simulink model "RLcircuit"  (R2018a)
settings: Solver=ode45  StartTime=0.0  StopTime=5.0  RelTol=1e-3
values from neighbouring files (symbols this model uses):
  R = sqrt(x.^2+y.^2)    [ex2_5.m]
undefined symbols (not defined in the file or in its folder): L
settings Model: Creator=Guestmit  LastModifiedBy=Guestmit

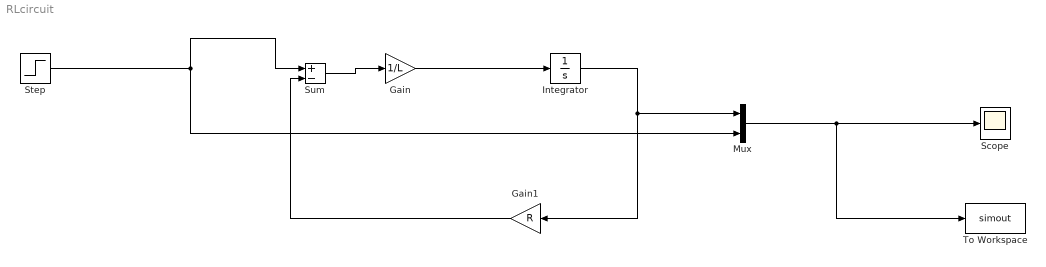
== system RLcircuit ==
  Gain : Gain  Gain=1/L
  Gain1 : Gain  Gain=R
  Integrator : Integrator
  Mux : Mux  Inputs=2
  Scope : Scope
  Step : Step  SampleTime=0
  Sum : Sum  Inputs=+-
  To Workspace : ToWorkspace  VariableName=simout  SaveFormat=Timeseries  SampleTime=-1
  wires:
  Step/1 -> Mux/2, Sum/1
  Sum/1 -> Gain/1
  Gain/1 -> Integrator/1
  Integrator/1 -> Gain1/1, Mux/1
  Gain1/1 -> Sum/2
  Mux/1 -> Scope/1, To Workspace/1
